simulink model "pwm"  (R2021a)
settings: Solver=VariableStepAuto  StartTime=0.0  StopTime=1  RelTol=1e-3
settings Model: Creator=simut  LastModifiedBy=simut

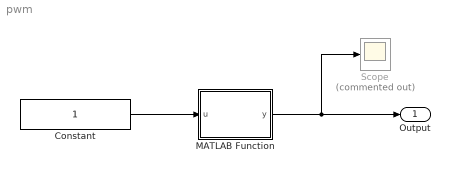
== system pwm ==
  Constant : Constant
  MATLAB Function : MATLAB Function  TreatAsAtomicUnit=on
  Scope : Scope  Commented=on
  Output : Outport
  wires:
  Constant/1 -> MATLAB Function/1(u)
  MATLAB Function/1(y) -> Scope/1, Output/1

== matlab function pwm/MATLAB Function ==
  data: u input; y output
function y = thrust_to_PWM(u)
    c0 = 32602.48313930042;
    c1 = 2585.2268555381825;
    y = c0 + c1*u;
